simulink model "vehicle"  (R2015b)
settings: Solver=ode3  SolverMode=SingleTasking  StartTime=0.0  StopTime=10.0  FixedStep=0.005  RelTol=1e-3
settings Model: Creator=Josef  LastModifiedBy=Josef
settings DataIOCC: SaveFormat=Array
settings OptimizationCC: BlockReduction=off  BooleanDataType=off
settings DebuggingCC: SaveWithParameterizedLinksMsg=none  SignalResolutionControl=TryResolveAllWithWarning
settings HardwareCC: ProdBitPerPointer=32  ProdLargestAtomicFloat=None  ProdIntDivRoundTo=Undefined  ProdEndianess=Unspecified  ProdWordSize=32  ProdHWDeviceType=32-bit Generic  TargetUnknown=on
settings ModelReferenceCC: ModelReferenceMinAlgLoopOccurrences=on
settings GRTTargetCC: GeneratePreprocessorConditionals=Disable all
settings ConfigComp: CovModelRefEnable=Off  CovSFcnEnable=off

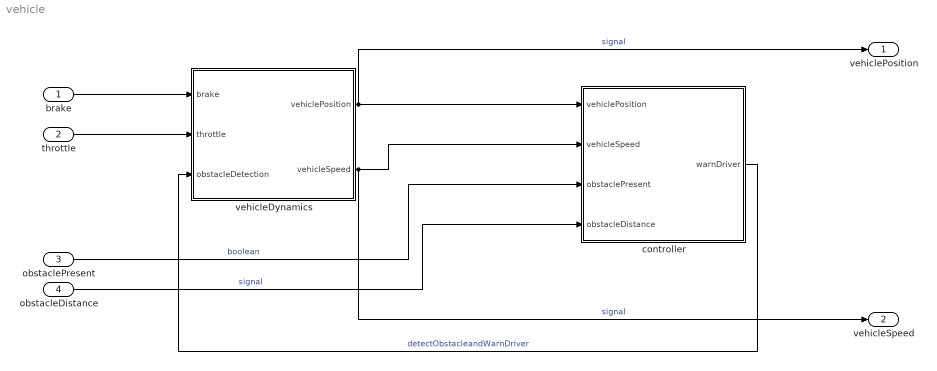
== system vehicle ==
  brake : Inport
  throttle : Inport  Port=2
  obstaclePresent : Inport  Port=3
      settings: AttributesFormatString=boolean
  obstacleDistance : Inport  Port=4
      settings: AttributesFormatString=signal
  controller : Subsystem
      settings: AttributesFormatString=CWS
  vehicleDynamics : Subsystem
  vehiclePosition : Outport
      settings: AttributesFormatString=signal
  vehicleSpeed : Outport  Port=2
      settings: AttributesFormatString=signal
  wires:
  vehicleDynamics/1(vehiclePosition) -> vehiclePosition/1, controller/1(vehiclePosition)  "signal"
  vehicleDynamics/2(vehicleSpeed) -> vehicleSpeed/1, controller/2(vehicleSpeed)  "signal"
  controller/1(warnDriver) -> vehicleDynamics/3(obstacleDetection)  "detectObstacleandWarnDriver"
  obstacleDistance/1 -> controller/4(obstacleDistance)  "signal"
  obstaclePresent/1 -> controller/3(obstaclePresent)  "boolean"
  throttle/1 -> vehicleDynamics/2(throttle)
  brake/1 -> vehicleDynamics/1(brake)

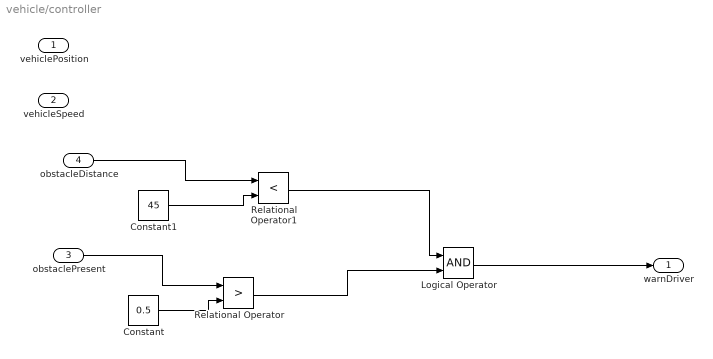
== system vehicle/controller ==
  vehiclePosition : Inport
      settings: AttributesFormatString=signal
  vehicleSpeed : Inport  Port=2
      settings: AttributesFormatString=signal
  obstaclePresent : Inport  Port=3
      settings: AttributesFormatString=boolean
  obstacleDistance : Inport  Port=4
      settings: AttributesFormatString=signal
  Constant : Constant  Value=0.5
  Constant1 : Constant  Value=45
  Logical Operator : Logic  AllPortsSameDT=off  OutDataTypeStr=boolean
  Relational Operator : RelationalOperator  Operator=>  OutDataTypeStr=boolean
  Relational Operator1 : RelationalOperator  Operator=<  OutDataTypeStr=boolean
  warnDriver : Outport
      settings: AttributesFormatString=detectObstacleandWarnDriver
  wires:
  Constant/1 -> Relational Operator/2
  obstaclePresent/1 -> Relational Operator/1
  obstacleDistance/1 -> Relational Operator1/1
  Constant1/1 -> Relational Operator1/2
  Relational Operator1/1 -> Logical Operator/1
  Relational Operator/1 -> Logical Operator/2
  Logical Operator/1 -> warnDriver/1

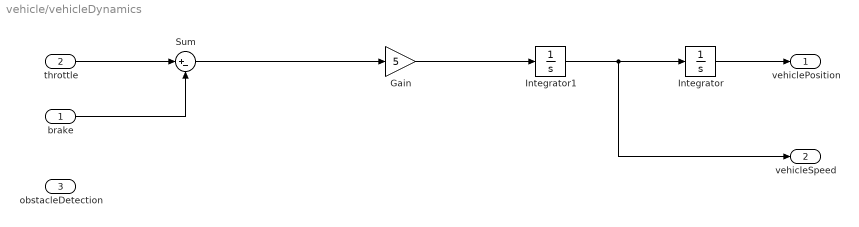
== system vehicle/vehicleDynamics ==
  brake : Inport
  throttle : Inport  Port=2
  obstacleDetection : Inport  Port=3
      settings: AttributesFormatString=detectObstacleandWarnDriver
  Gain : Gain  Gain=5
  Integrator : Integrator
  Integrator1 : Integrator
  Sum : Sum  Inputs=|+-
  vehiclePosition : Outport
      settings: AttributesFormatString=signal
  vehicleSpeed : Outport  Port=2
      settings: AttributesFormatString=signal
  wires:
  Integrator/1 -> vehiclePosition/1
  Integrator1/1 -> vehicleSpeed/1, Integrator/1
  Gain/1 -> Integrator1/1
  Sum/1 -> Gain/1
  throttle/1 -> Sum/1
  brake/1 -> Sum/2
